simulink model "FOC_orginal"  (R2023b)
settings: Solver=FixedStepDiscrete  StartTime=0.0  StopTime=2  FixedStep=0.000001  RelTol=1e-3
libraries: simulink x2, spsDCVoltageSourceLib x1, spsPermanentMagnetSynchronousMachineLib x1, spsTwoLevelConverterLib x1, sps_lib x1
settings Model: Creator=18575  LastModifiedBy=Administrator

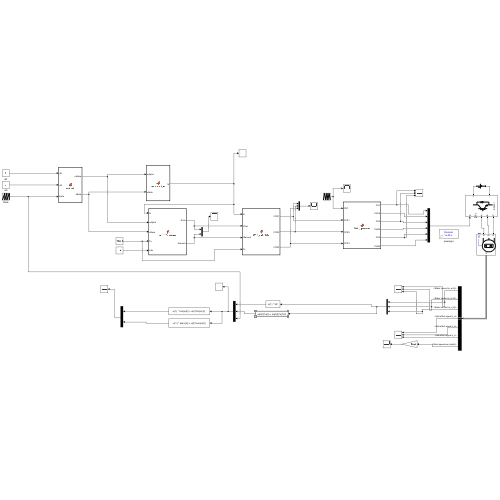
[thumbnail: Simulink's stored preview of the top-level diagram]
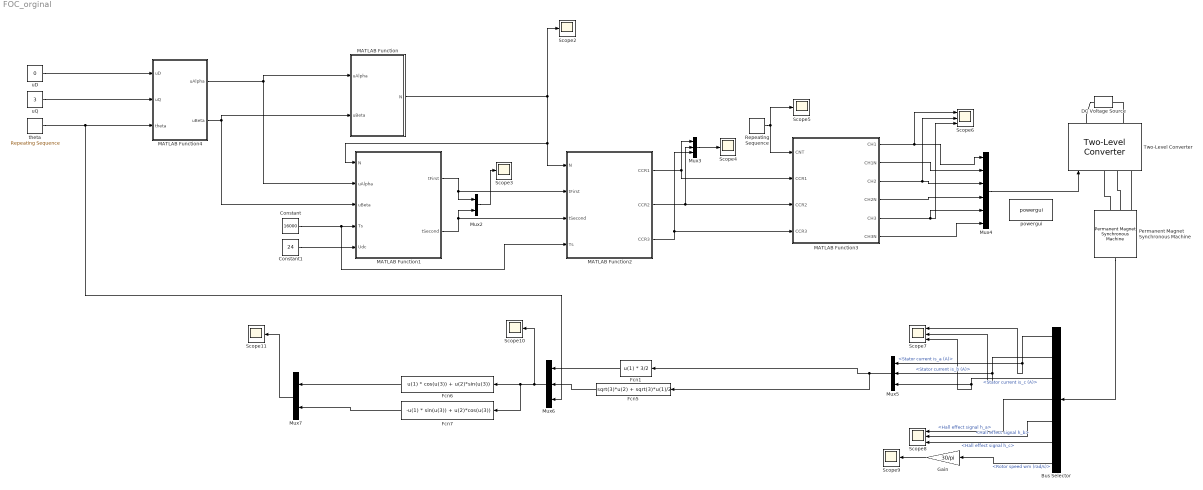
== system FOC_orginal ==
  Bus Selector : BusSelector  OutputSignals=Stator current is_a (A),Stator current is_b (A),Stator current is_c (A),Hall effect signal h_a,Hall effect signal h_b,Hall effect signal h_c,Rotor speed wm (rad/s)
  Constant : Constant  Value=16000
  Constant1 : Constant  Value=24
  DC Voltage Source : spsDCVoltageSourceLib/DC Voltage Source  Amplitude=24  Measurements=None
  Fcn1 : Fcn  Expr=u(1) * 3/2
  Fcn5 : Fcn  Expr=sqrt(3)*u(2) + sqrt(3)*u(1)/2
  Fcn6 : Fcn  Expr=u(1) * cos(u(3)) + u(2)*sin(u(3))
  Fcn7 : Fcn  Expr=-u(1) * sin(u(3)) + u(2)*cos(u(3))
  Gain : Gain  Gain=30/pi
  MATLAB Function : MATLAB Function  TreatAsAtomicUnit=on
  MATLAB Function1 : MATLAB Function  TreatAsAtomicUnit=on
  MATLAB Function2 : MATLAB Function  TreatAsAtomicUnit=on
  MATLAB Function3 : MATLAB Function  TreatAsAtomicUnit=on
  MATLAB Function4 : MATLAB Function  TreatAsAtomicUnit=on
  Mux2 : Mux  Inputs=2
  Mux3 : Mux  Inputs=3
  Mux4 : Mux  Inputs=6
  Mux5 : Mux  Inputs=3
  Mux6 : Mux  Inputs=3
  Mux7 : Mux  Inputs=2
  Permanent Magnet Synchronous Machine : spsPermanentMagnetSynchronousMachineLib/Permanent Magnet Synchronous Machine  NbPhases=3  FluxDistribution=Sinusoidal  RotorType=Round  MechanicalLoad=Torque Tm  PresetModel=No  ShowDetailedParameters=on  MeasurementBus=off  Resistance=0.0485  Inductance=8.5e-3  dqInductances=[8.5e-3,8.5e-3]  La=0.000395  MachineConstant=Flux linkage established by magnets (V.s)  Flux=0.1194  VoltageCst=43.3135  TorqueCst=0.3582  Flat=120  Mechanical=[0.0027 0.0004924 2 0]  PolePairs=4  InitialConditions=[0,0, 0,0]  InitialConditions5ph=[0 0 0 0 0 0]  RefAngle=Aligned with phase A axis (original Park)  IterativeDiscreteModel=Trapezoidal non iterative  TsBlock=-1  TsPowergui=0
  Repeating Sequence : simulink/Sources/Repeating Sequence  rep_seq_t=[0 0.00005 0.0001]  rep_seq_y=[0 8000 0]
  Scope{2..5,9..11} (7 alike) : Scope
  Scope6 : Scope  NumInputPorts=3
  Scope7 : Scope  NumInputPorts=3
  Scope8 : Scope  NumInputPorts=3
  Two-Level Converter : spsTwoLevelConverterLib/Two-Level Converter  ModelType=Switching devices  Ron=1e-3  Rs=1e6  Cs=inf  Vforward=[0,0]  Ron_Diode=1e-3  Rs_Diode=1e6  Cs_Diode=inf  Vf_Diode=1e-3  Rs_CurrentSource=inf  Ron_ACsource=1e-3
      settings: LibrarySourceBlock=sps_lib/Power Electronics/Two-Level Converter
  powergui : sps_lib/powergui  Priority=1  SimulationMode=Discrete  SampleTime=0.000001  frequency=60  Iterations=50  frequencyindice=0  Pbase=100e6  ErrMax=1e-4  UnitsV=kV  UnitsW=MW  buscounter=0  FunctionMessages=off  echomessages=off  EnableUseOfTLC=off  CurrentSourceSwitches=off  DisableSnubberDevices=off  DisableRonSwitches=off  DisableVfSwitches=off  DisplayEquations=off  AutomaticDiscreteSolvers=off  SolverType=Tustin/Backward Euler (TBE)  Interpol=off  ExternalGateDelay=off  methode=off  Ts=100  x0status=blocks  SPID=on  SwTol=0  HookPort=off  NonlinearTolerance=1e-4  nMaxIteration=100  ContinueOnMaxIteration=off  RestoreLinks=warning  ResistiveCurrentMeasurement=off  Frange=[0:2:500]  Ylog=off  Xlog=on  ShowGrid=off  save=off  variable=ZData  structure=0  ZoomFFT=off  StartTime=0.0  cycles=1  DisplayStyle=1  fundamental=60  FreqAxis=off  MaxFrequency=1000  frequencyindicesteady=1  RmsSteady=1  display=off
  "theta " : simulink/Sources/Repeating Sequence  rep_seq_t=[0 0.5]  rep_seq_y=[0 2*pi]
  uD : Constant  Value=0
  uQ : Constant  Value=3
  wires:
  uQ/1 -> MATLAB Function4/2(uQ)
  uD/1 -> MATLAB Function4/1(uD)
  "theta "/1 -> Mux6/3, MATLAB Function4/3(theta)
  MATLAB Function/1(N) -> Scope2/1, MATLAB Function1/1(N), MATLAB Function2/1(N)
  Constant/1 -> MATLAB Function2/4(Ts), MATLAB Function1/4(Ts)
  Constant1/1 -> MATLAB Function1/5(Udc)
  MATLAB Function1/1(tFirst) -> MATLAB Function2/2(tFirst), Mux2/1
  MATLAB Function1/2(tSecond) -> MATLAB Function2/3(tSecond), Mux2/2
  Mux2/1 -> Scope3/1
  MATLAB Function2/2(CCR2) -> Mux3/2, MATLAB Function3/3(CCR2)
  MATLAB Function2/1(CCR1) -> MATLAB Function3/2(CCR1), Mux3/1
  MATLAB Function2/3(CCR3) -> Mux3/3, MATLAB Function3/4(CCR3)
  Mux3/1 -> Scope4/1
  Repeating Sequence/1 -> Scope5/1, MATLAB Function3/1(CNT)
  MATLAB Function3/3(CH2) -> Scope6/2, Mux4/3
  MATLAB Function3/4(CH2N) -> Mux4/4
  MATLAB Function3/2(CH1N) -> Mux4/2
  MATLAB Function3/5(CH3) -> Scope6/3, Mux4/5
  MATLAB Function3/1(CH1) -> Scope6/1, Mux4/1
  MATLAB Function3/6(CH3N) -> Mux4/6
  Mux4/1 -> Two-Level Converter/1
  Permanent Magnet Synchronous Machine/1 -> Bus Selector/1
  Bus Selector/1 -> Scope7/1, Mux5/1  "<Stator current is_a (A)>"
  Bus Selector/2 -> Scope7/2, Mux5/2  "<Stator current is_b (A)>"
  Bus Selector/3 -> Scope7/3, Mux5/3  "<Stator current is_c (A)>"
  Bus Selector/4 -> Scope8/1  "<Hall effect signal h_a>"
  Bus Selector/5 -> Scope8/2  "<Hall effect signal h_b>"
  Bus Selector/6 -> Scope8/3  "<Hall effect signal h_c>"
  Bus Selector/7 -> Gain/1  "<Rotor speed wm (rad/s)>"
  Gain/1 -> Scope9/1
  Mux5/1 -> Fcn5/1, Fcn1/1
  Fcn1/1 -> Mux6/1
  Fcn5/1 -> Mux6/2
  Mux6/1 -> Fcn7/1, Fcn6/1, Scope10/1
  Fcn6/1 -> Mux7/1
  Fcn7/1 -> Mux7/2
  Mux7/1 -> Scope11/1
  MATLAB Function4/1(uAlpha) -> MATLAB Function1/2(uAlpha), MATLAB Function/1(uAlpha)
  MATLAB Function4/2(uBeta) -> MATLAB Function1/3(uBeta), MATLAB Function/2(uBeta)
  connections:
  Two-Level Converter/RConn1 -- DC Voltage Source/RConn1
  Two-Level Converter/RConn2 -- DC Voltage Source/LConn1
  Permanent Magnet Synchronous Machine/LConn3 -- Two-Level Converter/LConn3
  Permanent Magnet Synchronous Machine/LConn1 -- Two-Level Converter/LConn1
  Permanent Magnet Synchronous Machine/LConn2 -- Two-Level Converter/LConn2

== matlab function FOC_orginal/MATLAB Function1 ==
  data: N input; tFirst output; uAlpha input; uBeta input; tSecond output; Ts input; Udc input
function [tFirst, tSecond] = vectorCalculate(N, uAlpha, uBeta, Ts, Udc)

tFirst = 0;
tSecond = 0;

X = sqrt(3)*Ts*uBeta/Udc;
Y = sqrt(3)*Ts/Udc*(sqrt(3)*uAlpha/2+uBeta/2);
Z = sqrt(3)*Ts/Udc*(-sqrt(3)*uAlpha/2+uBeta/2);

if (N == 1)
    tFirst = Z;
    tSecond = Y;
end

if (N==2)
    tFirst = Y;
    tSecond = -X;
end

if (N==3)
    tFirst =-Z;
    tSecond = X;
end

if (N==4)
    tFirst =-X;
    tSecond = Z;
end

if (N==5)
    tFirst =X;
    tSecond = -Y;
end

if (N==6)
    tFirst =-Y;
    tSecond = -Z;
end

== matlab function FOC_orginal/MATLAB Function ==
  data: uAlpha input; N output; uBeta input

function N = sectorJudge(uAlpha, uBeta)

u1 = uBeta;
u2 = sqrt(3)/2*uAlpha - 1/2*uBeta;
u3 = -sqrt(3)/2*uAlpha - 1/2*uBeta;

N = 0;
if (u1 > 0)
    N = N+1;
end;

if (u2 > 0)
    N = N+2;
end;

if (u3 > 0)
    N = N+4;
end;

== matlab function FOC_orginal/MATLAB Function2 ==
  data: N input; CCR1 output; tFirst input; tSecond input; CCR2 output; Ts input; CCR3 output
function [CCR1, CCR2, CCR3] =  CCR_calculate(N, tFirst, tSecond,  Ts)

CCR1 = 0;
CCR2 = 0;
CCR3 = 0;

t = tFirst + tSecond;
if (t > Ts)
    tFirst = tFirst/t * Ts;
    tSecond = tSecond / t * Ts;
end

value1 = (Ts - tFirst - tSecond) /4;  % vector 0 or 7 
value2 = value1 + tFirst / 2;
value3 = value2 + tSecond / 2;

switch(N)
    case 3
        CCR1 = value1;
        CCR2 = value2;
        CCR3 = value3;

    case 1
        CCR1 = value2;
        CCR2 = value1;
        CCR3 = value3;

    case 5
        CCR1 = value3;
        CCR2 = value1;
        CCR3 = value2;

    case 4
        CCR1 = value3;
        CCR2 = value2;
        CCR3 = value1;

    case 6
        CCR1 = value2;
        CCR2 = value3;
        CCR3 = value1;

    case 2
        CCR1 = value1;
        CCR2 = value3;
        CCR3 = value2;

end

== matlab function FOC_orginal/MATLAB Function3 ==
  data: CNT input; CH1 output; CCR1 input; CCR2 input; CH1N output; CCR3 input; CH2 output; CH2N output; CH3 output; CH3N output
function [CH1, CH1N, CH2, CH2N,CH3, CH3N] =  PWM_generate(CNT,CCR1, CCR2,  CCR3)

CH1 = 0;
CH1N = 0;
CH2 = 0;
CH2N = 0;
CH3 = 0;
CH3N = 0;

if (CNT > CCR1)
    CH1 = 1;
    CH1N = 0;
else
    CH1 = 0;
    CH1N = 1;
end

if (CNT > CCR2)
    CH2 = 1;
    CH2N = 0;
else
    CH2 = 0;
    CH2N = 1;
end


if (CNT > CCR3)
    CH3 = 1;
    CH3N = 0;
else
    CH3 = 0;
    CH3N = 1;
end

== matlab function FOC_orginal/MATLAB Function4 ==
  data: uD input; uAlpha output; uQ input; theta input; uBeta output
function [uAlpha, uBeta] = revPark(uD, uQ, theta)


uAlpha = 0;
uBeta = 0;

uAlpha = cos(theta) * uD - sin(theta) *uQ;
uBeta = sin(theta) * uD + cos(theta) * uQ;
